simulink model "OpenMan"  (R2018a)
settings: Solver=ode5  StartTime=0.0  StopTime=T  FixedStep=0.02  RelTol=1e-3
undefined symbols (not defined in the file or in its folder): Base, Link1, Link2, Link3, Link4, OpenMan, RootPart
libraries: mblibv1 x18, simulink x4
settings Model: Creator=Administrator  LastModifiedBy=Hungs
settings CodeAppCC: StateflowObjectComments=on
settings SimscapeCC: SimscapeNormalizeSystem=off
settings SimMechanicsCC: VisOnUpdateDiagram=on  VisDuringSimulation=on

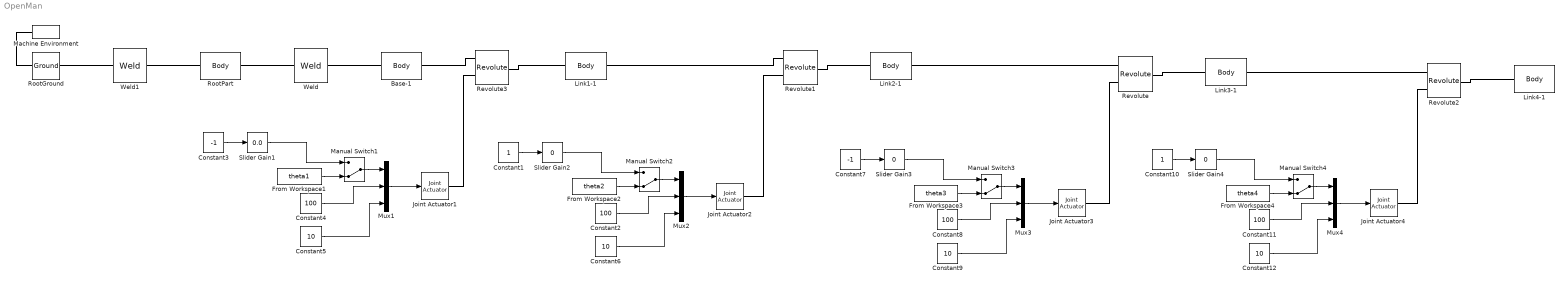
== system OpenMan ==
  Base-1 : mblibv1/Bodies/Body  LConnTagsString=CS2  RConnTagsString=CS3  UpdateFromCAD=on  PMImportedID=Base-1  DialogClass=MechanicalBodyBlock  Mass=0.0428629  MassUnits=kg  InertiaUnits=kg*m^2  Inertia=[6.81332e-06,0,-9.39051e-08;0,1.19906e-05,0;-9.39051e-08,0,1.05921e-05]  Shape=Cylinder  ShapeDims=[1 1]  ShapeUnits=m  ShapeUse=false  Density=1  DensityUnits=kg/m^3  DensityUse=false  GraphicsMode=GFXFILE  GraphicsFileName=OpenMan - Base-1.STL  BodyColorSelMode=COLORPALETTE  BodyColor=[0.64706;0.61961;0.58823]  AttachedToCS=CS1  CG=Right$CG$[-0.0116952 0 0.017999]$WORLD$WORLD$m$[1 0 0;0 1 0;0 0 1]$3x3 Transform$rad$WORLD$false$Base-1::CG(AUTOGEN)  WorkingFrames=Right$CS1$[0 0 0]$WORLD$WORLD$m$[1 0 0;0 1 0;0 0 1]$3x3 Transform$rad$WORLD$false$Base-1::CS1(AUTOGEN)#Left$CS2$[-0.0116952 0 0.017999]$WORLD$WORLD$m$[1 0 0;0 1 0;0 0 1]$3x3 Transform$rad$WORLD$true$Base-1:-:OpenMan/RootPart::Base-1(AUTOGEN)#Right$CS3$[0 0 0.036]$WORLD$WORLD$m$[1 0 0;0 1 0;0 0 1]$3x3 Transform$rad$WORLD$true$Base-1:-:Link1-1::Base-1(AUTOGEN)  CGPos=[-0.0116952 0 0.017999]  CGRot=[1 0 0;0 1 0;0 0 1]  CS0Pos=[]  CS0Rot=[]  CS1Pos=[0 0 0]  CS1Rot=[1 0 0;0 1 0;0 0 1]  CS2Pos=[-0.0116952 0 0.017999]  CS2Rot=[1 0 0;0 1 0;0 0 1]  CS3Pos=[0 0 0.036]  CS3Rot=[1 0 0;0 1 0;0 0 1]  CS4Pos=[]  CS4Rot=[]  CS5Pos=[]  CS5Rot=[]  CS6Pos=[]  CS6Rot=[]  CS7Pos=[]  CS7Rot=[]  CS8Pos=[]  CS8Rot=[]  CS9Pos=[]  CS9Rot=[]  CS10Pos=[]  CS10Rot=[]  CS11Pos=[]  CS11Rot=[]  CS12Pos=[]  CS12Rot=[]  CS13Pos=[]  CS13Rot=[]  CS14Pos=[]  CS14Rot=[]  CS15Pos=[]  CS15Rot=[]  CS16Pos=[]  CS16Rot=[]  CS17Pos=[]  CS17Rot=[]  CS18Pos=[]  CS18Rot=[]  CS19Pos=[]  CS19Rot=[]  CS20Pos=[]  CS20Rot=[]
      settings: SourceProductName=Simscape Multibody  SourceProductBaseCode=MS
  Constant1 : Constant
  Constant10 : Constant
  Constant{2,4,8,11} (4 alike) : Constant  Value=100
  Constant{5..6,9,12} (4 alike) : Constant  Value=10
  Constant3 : Constant  Value=-1
  Constant7 : Constant  Value=-1
  From Workspace1 : FromWorkspace  VariableName=theta1  SampleTime=0  OutputAfterFinalValue=Holding final value
  From Workspace2 : FromWorkspace  VariableName=theta2  SampleTime=0  OutputAfterFinalValue=Holding final value
  From Workspace3 : FromWorkspace  VariableName=theta3  SampleTime=0  OutputAfterFinalValue=Holding final value
  From Workspace4 : FromWorkspace  VariableName=theta4  SampleTime=0  OutputAfterFinalValue=Holding final value
  Joint Actuator{1..4} (4 alike) : mblibv1/Sensors &  Actuators/Joint Actuator  UpdateFromCAD=off  PhysicalDomain=Mechanical  PortType=blob  ActuationStyle=Motion  AngleUnits=deg  ArcVelocityUnits=deg/s  ArcAccelerationUnits=deg/s^2  CoordPositionUnits=m  VelocityUnits=m/s  AccelerationUnits=m/s^2  ForceUnits=N  TorqueUnits=N*m  ActiveIO=on  Width=3  DialogClass=MechanicalActuatorBlock  Primitive=R1  ReferenceFrame=Absolute (World)
      settings: SourceProductName=Simscape  SourceProductBaseCode=SS
  Link1-1 : mblibv1/Bodies/Body  LConnTagsString=CS3  RConnTagsString=CS2  UpdateFromCAD=on  PMImportedID=Link1-1  DialogClass=MechanicalBodyBlock  Mass=0.0553342  MassUnits=kg  InertiaUnits=kg*m^2  Inertia=[1.8235e-05,0,0;0,1.05975e-05,0;0,0,1.53152e-05]  Shape=Cylinder  ShapeDims=[1 1]  ShapeUnits=m  ShapeUse=false  Density=1  DensityUnits=kg/m^3  DensityUse=false  GraphicsMode=GFXFILE  GraphicsFileName=OpenMan - Link1-1.STL  BodyColorSelMode=COLORPALETTE  BodyColor=[0;1;0]  AttachedToCS=CS1  CG=Right$CG$[0 0 0.05625]$WORLD$WORLD$m$[1 0 0;0 0 -1;0 1 0]$3x3 Transform$rad$WORLD$false$Link1-1::CG(AUTOGEN)  WorkingFrames=Right$CS1$[0 0 0.0765]$WORLD$WORLD$m$[1 0 0;0 0 -1;0 1 0]$3x3 Transform$rad$WORLD$false$Link1-1::CS1(AUTOGEN)#Right$CS2$[0 0.019 0.0765]$WORLD$WORLD$m$[1 0 0;0 1 0;0 0 1]$3x3 Transform$rad$WORLD$true$Link1-1:-:Link2-1::Link1-1(AUTOGEN)#Left$CS3$[0 0 0.036]$WORLD$WORLD$m$[1 0 0;0 1 0;0 0 1]$3x3 Transform$rad$WORLD$true$Base-1:-:Link1-1::Link1-1(AUTOGEN)  CGPos=[0 0 0.05625]  CGRot=[1 0 0;0 0 -1;0 1 0]  CS0Pos=[]  CS0Rot=[]  CS1Pos=[0 0 0.0765]  CS1Rot=[1 0 0;0 0 -1;0 1 0]  CS2Pos=[0 0.019 0.0765]  CS2Rot=[1 0 0;0 1 0;0 0 1]  CS3Pos=[0 0 0.036]  CS3Rot=[1 0 0;0 1 0;0 0 1]  CS4Pos=[]  CS4Rot=[]  CS5Pos=[]  CS5Rot=[]  CS6Pos=[]  CS6Rot=[]  CS7Pos=[]  CS7Rot=[]  CS8Pos=[]  CS8Rot=[]  CS9Pos=[]  CS9Rot=[]  CS10Pos=[]  CS10Rot=[]  CS11Pos=[]  CS11Rot=[]  CS12Pos=[]  CS12Rot=[]  CS13Pos=[]  CS13Rot=[]  CS14Pos=[]  CS14Rot=[]  CS15Pos=[]  CS15Rot=[]  CS16Pos=[]  CS16Rot=[]  CS17Pos=[]  CS17Rot=[]  CS18Pos=[]  CS18Rot=[]  CS19Pos=[]  CS19Rot=[]  CS20Pos=[]  CS20Rot=[]
      settings: SourceProductName=Simscape Multibody  SourceProductBaseCode=MS
  Link2-1 : mblibv1/Bodies/Body  LConnTagsString=CS3  RConnTagsString=CS2  UpdateFromCAD=on  PMImportedID=Link2-1  DialogClass=MechanicalBodyBlock  Mass=0.117048  MassUnits=kg  InertiaUnits=kg*m^2  Inertia=[0.000233359,-2.83101e-05,0;-2.83101e-05,3.2542e-05,0;0,0,0.00023539]  Shape=Cylinder  ShapeDims=[1 1]  ShapeUnits=m  ShapeUse=false  Density=1  DensityUnits=kg/m^3  DensityUse=false  GraphicsMode=GFXFILE  GraphicsFileName=OpenMan - Link2-1.STL  BodyColorSelMode=COLORPALETTE  BodyColor=[1;1;0]  AttachedToCS=CS1  CG=Right$CG$[0.012 0 0.1405]$WORLD$WORLD$m$[1 0 0;0 0 -1;0 1 0]$3x3 Transform$rad$WORLD$false$Link2-1::CG(AUTOGEN)  WorkingFrames=Right$CS1$[0.024 0 0.2045]$WORLD$WORLD$m$[1 0 0;0 0 -1;0 1 0]$3x3 Transform$rad$WORLD$false$Link2-1::CS1(AUTOGEN)#Right$CS2$[0.024 -0.019 0.2045]$WORLD$WORLD$m$[1 0 0;0 1 0;0 0 1]$3x3 Transform$rad$WORLD$true$Link2-1:-:Link3-1::Link2-1(AUTOGEN)#Left$CS3$[0 0.019 0.0765]$WORLD$WORLD$m$[1 0 0;0 1 0;0 0 1]$3x3 Transform$rad$WORLD$true$Link1-1:-:Link2-1::Link2-1(AUTOGEN)  CGPos=[0.012 0 0.1405]  CGRot=[1 0 0;0 0 -1;0 1 0]  CS0Pos=[]  CS0Rot=[]  CS1Pos=[0.024 0 0.2045]  CS1Rot=[1 0 0;0 0 -1;0 1 0]  CS2Pos=[0.024 -0.019 0.2045]  CS2Rot=[1 0 0;0 1 0;0 0 1]  CS3Pos=[0 0.019 0.0765]  CS3Rot=[1 0 0;0 1 0;0 0 1]  CS4Pos=[]  CS4Rot=[]  CS5Pos=[]  CS5Rot=[]  CS6Pos=[]  CS6Rot=[]  CS7Pos=[]  CS7Rot=[]  CS8Pos=[]  CS8Rot=[]  CS9Pos=[]  CS9Rot=[]  CS10Pos=[]  CS10Rot=[]  CS11Pos=[]  CS11Rot=[]  CS12Pos=[]  CS12Rot=[]  CS13Pos=[]  CS13Rot=[]  CS14Pos=[]  CS14Rot=[]  CS15Pos=[]  CS15Rot=[]  CS16Pos=[]  CS16Rot=[]  CS17Pos=[]  CS17Rot=[]  CS18Pos=[]  CS18Rot=[]  CS19Pos=[]  CS19Rot=[]  CS20Pos=[]  CS20Rot=[]
      settings: SourceProductName=Simscape Multibody  SourceProductBaseCode=MS
  Link3-1 : mblibv1/Bodies/Body  LConnTagsString=CS2  RConnTagsString=CS3  UpdateFromCAD=on  PMImportedID=Link3-1  DialogClass=MechanicalBodyBlock  Mass=0.0869839  MassUnits=kg  InertiaUnits=kg*m^2  Inertia=[1.69409e-05,0,0;0,0.000140539,0;0,0,0.000129904]  Shape=Cylinder  ShapeDims=[1 1]  ShapeUnits=m  ShapeUse=false  Density=1  DensityUnits=kg/m^3  DensityUse=false  GraphicsMode=GFXFILE  GraphicsFileName=OpenMan - Link3-1.STL  BodyColorSelMode=COLORPALETTE  BodyColor=[0;0;1]  AttachedToCS=CS1  CG=Right$CG$[0.086 0 0.2045]$WORLD$WORLD$m$[1 0 0;0 0 -1;0 1 0]$3x3 Transform$rad$WORLD$false$Link3-1::CG(AUTOGEN)  WorkingFrames=Right$CS1$[0.148 0 0.2045]$WORLD$WORLD$m$[1 0 0;0 0 -1;0 1 0]$3x3 Transform$rad$WORLD$false$Link3-1::CS1(AUTOGEN)#Left$CS2$[0.024 -0.019 0.2045]$WORLD$WORLD$m$[1 0 0;0 1 0;0 0 1]$3x3 Transform$rad$WORLD$true$Link2-1:-:Link3-1::Link3-1(AUTOGEN)#Right$CS3$[0.148 0.019 0.2045]$WORLD$WORLD$m$[1 0 0;0 1 0;0 0 1]$3x3 Transform$rad$WORLD$true$Link3-1:-:Link4-1::Link3-1(AUTOGEN)  CGPos=[0.086 0 0.2045]  CGRot=[1 0 0;0 0 -1;0 1 0]  CS0Pos=[]  CS0Rot=[]  CS1Pos=[0.148 0 0.2045]  CS1Rot=[1 0 0;0 0 -1;0 1 0]  CS2Pos=[0.024 -0.019 0.2045]  CS2Rot=[1 0 0;0 1 0;0 0 1]  CS3Pos=[0.148 0.019 0.2045]  CS3Rot=[1 0 0;0 1 0;0 0 1]  CS4Pos=[]  CS4Rot=[]  CS5Pos=[]  CS5Rot=[]  CS6Pos=[]  CS6Rot=[]  CS7Pos=[]  CS7Rot=[]  CS8Pos=[]  CS8Rot=[]  CS9Pos=[]  CS9Rot=[]  CS10Pos=[]  CS10Rot=[]  CS11Pos=[]  CS11Rot=[]  CS12Pos=[]  CS12Rot=[]  CS13Pos=[]  CS13Rot=[]  CS14Pos=[]  CS14Rot=[]  CS15Pos=[]  CS15Rot=[]  CS16Pos=[]  CS16Rot=[]  CS17Pos=[]  CS17Rot=[]  CS18Pos=[]  CS18Rot=[]  CS19Pos=[]  CS19Rot=[]  CS20Pos=[]  CS20Rot=[]
      settings: SourceProductName=Simscape Multibody  SourceProductBaseCode=MS
  Link4-1 : mblibv1/Bodies/Body  LConnTagsString=CS2  UpdateFromCAD=on  PMImportedID=Link4-1  DialogClass=MechanicalBodyBlock  Mass=0.16348  MassUnits=kg  InertiaUnits=kg*m^2  Inertia=[0.000112546,0,0;0,0.000266976,0;0,0,0.000183011]  Shape=Cylinder  ShapeDims=[1 1]  ShapeUnits=m  ShapeUse=false  Density=1  DensityUnits=kg/m^3  DensityUse=false  GraphicsMode=GFXFILE  GraphicsFileName=OpenMan - Link4-1.STL  BodyColorSelMode=COLORPALETTE  BodyColor=[1 0 0]  AttachedToCS=CS1  CG=Right$CG$[0.211 0 0.2045]$WORLD$WORLD$m$[1 0 0;0 0 -1;0 1 0]$3x3 Transform$rad$WORLD$false$Link4-1::CG(AUTOGEN)  WorkingFrames=Right$CS1$[0.274 0 0.2045]$WORLD$WORLD$m$[1 0 0;0 0 -1;0 1 0]$3x3 Transform$rad$WORLD$false$Link4-1::CS1(AUTOGEN)#Left$CS2$[0.148 0.019 0.2045]$WORLD$WORLD$m$[1 0 0;0 1 0;0 0 1]$3x3 Transform$rad$WORLD$true$Link3-1:-:Link4-1::Link4-1(AUTOGEN)  CGPos=[0.211 0 0.2045]  CGRot=[1 0 0;0 0 -1;0 1 0]  CS0Pos=[]  CS0Rot=[]  CS1Pos=[0.274 0 0.2045]  CS1Rot=[1 0 0;0 0 -1;0 1 0]  CS2Pos=[0.148 0.019 0.2045]  CS2Rot=[1 0 0;0 1 0;0 0 1]  CS3Pos=[]  CS3Rot=[]  CS4Pos=[]  CS4Rot=[]  CS5Pos=[]  CS5Rot=[]  CS6Pos=[]  CS6Rot=[]  CS7Pos=[]  CS7Rot=[]  CS8Pos=[]  CS8Rot=[]  CS9Pos=[]  CS9Rot=[]  CS10Pos=[]  CS10Rot=[]  CS11Pos=[]  CS11Rot=[]  CS12Pos=[]  CS12Rot=[]  CS13Pos=[]  CS13Rot=[]  CS14Pos=[]  CS14Rot=[]  CS15Pos=[]  CS15Rot=[]  CS16Pos=[]  CS16Rot=[]  CS17Pos=[]  CS17Rot=[]  CS18Pos=[]  CS18Rot=[]  CS19Pos=[]  CS19Rot=[]  CS20Pos=[]  CS20Rot=[]
      settings: SourceProductName=Simscape Multibody  SourceProductBaseCode=MS
  Machine Environment : mblibv1/Bodies/Machine Environment  PortType=env  PhysicalDomain=Mechanical  DialogTemplateClass=MECH.MachineEnvironment  SyncWhenCopied=off  Gravity=[0 -9.81 0]  GravityUnits=m/s^2  GravityAsSignal=off  Dimensionality=Auto-detect  AnalysisType=Forward dynamics  LinearAssemblyTolerance=1e-3  LinearAssemblyToleranceUnits=m  AngularAssemblyTolerance=1e-3  AngularAssemblyToleranceUnits=rad  ConstraintSolverType=Stabilizing  ConstraintRelTolerance=1e-4  ConstraintAbsTolerance=1e-4  UseRobustSingularityHandling=off  RedundancyAnalysisToleranceType=Automatically select tolerance  RedundancyAnalysisTolerance=1e-14  StatePerturbationType=Fixed  PerturbationSize=1e-5  VisualizeMachine=on  BodyVisualizationType=Use model default body geometries  BodyColorSelMode=Use model default  DefaultBodyColor=[1 0 0]
      settings: SourceProductName=Simscape Multibody  SourceProductBaseCode=MS
  Manual Switch{1..4} (4 alike) : ManualSwitch  CurrentSetting=0
  Mux{1..4} (4 alike) : Mux  Inputs=3
  Revolute : mblibv1/Joints/Revolute  LConnTagsString=__newl0|SA1  RConnTagsString=__newr0  UpdateFromCAD=on  PMImportedID=Link2-1:-:Link3-1  NumSAPorts=1  CutJoint=off  MarkAsCut=off  Primitives=prismatic  PrimitiveProps=R1$World$[0,1,0]$revolute  DialogClass=JointBlock  R1Axis=[0,1,0]
      settings: SourceProductName=Simscape Multibody  SourceProductBaseCode=MS
  Revolute1 : mblibv1/Joints/Revolute  LConnTagsString=__newl0|SA1  RConnTagsString=__newr0  UpdateFromCAD=on  PMImportedID=Link1-1:-:Link2-1  NumSAPorts=1  CutJoint=off  MarkAsCut=off  Primitives=prismatic  PrimitiveProps=R1$World$[0,-1,0]$revolute  DialogClass=JointBlock  R1Axis=[0,-1,0]
      settings: SourceProductName=Simscape Multibody  SourceProductBaseCode=MS
  Revolute2 : mblibv1/Joints/Revolute  LConnTagsString=__newl0|SA1  RConnTagsString=__newr0  UpdateFromCAD=on  PMImportedID=Link3-1:-:Link4-1  NumSAPorts=1  CutJoint=off  MarkAsCut=off  Primitives=prismatic  PrimitiveProps=R1$World$[0,-1,0]$revolute  DialogClass=JointBlock  R1Axis=[0,-1,0]
      settings: SourceProductName=Simscape Multibody  SourceProductBaseCode=MS
  Revolute3 : mblibv1/Joints/Revolute  LConnTagsString=__newl0|SA1  RConnTagsString=__newr0  UpdateFromCAD=on  PMImportedID=Base-1:-:Link1-1  NumSAPorts=1  CutJoint=off  MarkAsCut=off  Primitives=prismatic  PrimitiveProps=R1$World$[0,0,-1]$revolute  DialogClass=JointBlock  R1Axis=[0,0,-1]
      settings: SourceProductName=Simscape Multibody  SourceProductBaseCode=MS
  RootGround : mblibv1/Bodies/Ground  UpdateFromCAD=on  PMImportedID=RootGround  LeftPortType=env  RightPortType=workingframe  PhysicalDomain=Mechanical  DialogClass=GroundBlock  CoordPosition=[0.219004,-0.00655955,0.163625]  CoordPositionUnits=m  StateVectorMgrId=0  MachineId=[1 0]  ShowEnvPort=on  ParameterChecksum=[2384219016, 3002916829, 4077460786, 3927882011]  TopologyChecksum=[2459791412, 654682897, 3936132905, 4259893478]
      settings: SourceProductName=Simscape Multibody  SourceProductBaseCode=MS
  RootPart : mblibv1/Bodies/Body  LConnTagsString=CS3  RConnTagsString=CS2  UpdateFromCAD=on  PMImportedID=OpenMan/RootPart  DialogClass=MechanicalBodyBlock  Mass=0  MassUnits=kg  InertiaUnits=kg*m^2  Inertia=[0,0,0;0,0,0;0,0,0]  Shape=Cylinder  ShapeDims=[1 1]  ShapeUnits=m  ShapeUse=false  Density=1  DensityUnits=kg/m^3  DensityUse=false  GraphicsMode=MACHINE_DEFAULT  BodyColorSelMode=MACHINE_DEFAULT  BodyColor=[1;0;0]  AttachedToCS=CS1  CG=Right$CG$[0.219004 -0.00655955 0.163625]$WORLD$WORLD$m$[1 0 0;0 1 0;0 0 1]$3x3 Transform$rad$WORLD$false$OpenMan/RootPart::CG(AUTOGEN)  WorkingFrames=Right$CS1$[0 0 0]$WORLD$WORLD$m$[1 0 0;0 1 0;0 0 1]$3x3 Transform$rad$WORLD$false$OpenMan/RootPart::CS1(AUTOGEN)#Right$CS2$[-0.0116952 0 0.017999]$WORLD$WORLD$m$[1 0 0;0 1 0;0 0 1]$3x3 Transform$rad$WORLD$true$Base-1:-:OpenMan/RootPart::OpenMan/RootPart(AUTOGEN)#Left$CS3$[0.219004 -0.00655955 0.163625]$WORLD$WORLD$m$[1 0 0;0 1 0;0 0 1]$3x3 Transform$rad$WORLD$true$OpenMan/RootPart:-:RootGround::OpenMan/RootPart(AUTOGEN)  CGPos=[0.219004 -0.00655955 0.163625]  CGRot=[1 0 0;0 1 0;0 0 1]  CS0Pos=[]  CS0Rot=[]  CS1Pos=[0 0 0]  CS1Rot=[1 0 0;0 1 0;0 0 1]  CS2Pos=[-0.0116952 0 0.017999]  CS2Rot=[1 0 0;0 1 0;0 0 1]  CS3Pos=[0.219004 -0.00655955 0.163625]  CS3Rot=[1 0 0;0 1 0;0 0 1]  CS4Pos=[]  CS4Rot=[]  CS5Pos=[]  CS5Rot=[]  CS6Pos=[]  CS6Rot=[]  CS7Pos=[]  CS7Rot=[]  CS8Pos=[]  CS8Rot=[]  CS9Pos=[]  CS9Rot=[]  CS10Pos=[]  CS10Rot=[]  CS11Pos=[]  CS11Rot=[]  CS12Pos=[]  CS12Rot=[]  CS13Pos=[]  CS13Rot=[]  CS14Pos=[]  CS14Rot=[]  CS15Pos=[]  CS15Rot=[]  CS16Pos=[]  CS16Rot=[]  CS17Pos=[]  CS17Rot=[]  CS18Pos=[]  CS18Rot=[]  CS19Pos=[]  CS19Rot=[]  CS20Pos=[]  CS20Rot=[]
      settings: SourceProductName=Simscape Multibody  SourceProductBaseCode=MS
  Slider Gain1 : simulink/Math Operations/Slider Gain  gain=0.0  low=-180  high=180
  Slider Gain2 : simulink/Math Operations/Slider Gain  gain=0  low=-180  high=180
  Slider Gain3 : simulink/Math Operations/Slider Gain  gain=0  low=-180  high=180
  Slider Gain4 : simulink/Math Operations/Slider Gain  gain=0  low=-180  high=180
  Weld : mblibv1/Joints/Weld  LConnTagsString=__newl0  RConnTagsString=__newr0  UpdateFromCAD=on  PMImportedID=Base-1:-:OpenMan/RootPart  NumSAPorts=0  CutJoint=off  MarkAsCut=off  Primitives=weld  PrimitiveProps=W$WORLD$[0.57735,0.57735,0.57735]$weld  DialogClass=JointBlock  WAxis=[0.57735,0.57735,0.57735]
      settings: SourceProductName=Simscape Multibody  SourceProductBaseCode=MS
  Weld1 : mblibv1/Joints/Weld  LConnTagsString=__newl0  RConnTagsString=__newr0  UpdateFromCAD=on  PMImportedID=OpenMan/RootPart:-:RootGround  NumSAPorts=0  CutJoint=off  MarkAsCut=off  Primitives=weld  PrimitiveProps=W$WORLD$[0.57735,0.57735,0.57735]$weld  DialogClass=JointBlock  WAxis=[0.57735,0.57735,0.57735]
      settings: SourceProductName=Simscape Multibody  SourceProductBaseCode=MS
  wires:
  Slider Gain1/1 -> Manual Switch1/1
  Manual Switch1/1 -> Mux1/1
  Constant3/1 -> Slider Gain1/1
  From Workspace1/1 -> Manual Switch1/2
  Constant5/1 -> Mux1/3
  Mux1/1 -> Joint Actuator1/1
  Constant4/1 -> Mux1/2
  Constant2/1 -> Mux2/2
  Manual Switch2/1 -> Mux2/1
  Constant6/1 -> Mux2/3
  Constant1/1 -> Slider Gain2/1
  From Workspace2/1 -> Manual Switch2/2
  Mux2/1 -> Joint Actuator2/1
  Slider Gain2/1 -> Manual Switch2/1
  Constant8/1 -> Mux3/2
  Manual Switch3/1 -> Mux3/1
  Constant9/1 -> Mux3/3
  Constant7/1 -> Slider Gain3/1
  From Workspace3/1 -> Manual Switch3/2
  Mux3/1 -> Joint Actuator3/1
  Slider Gain3/1 -> Manual Switch3/1
  Constant11/1 -> Mux4/2
  Manual Switch4/1 -> Mux4/1
  Constant12/1 -> Mux4/3
  Constant10/1 -> Slider Gain4/1
  From Workspace4/1 -> Manual Switch4/2
  Mux4/1 -> Joint Actuator4/1
  Slider Gain4/1 -> Manual Switch4/1
  connections:
  RootPart/RConn1 -- Weld/LConn1
  Weld/RConn1 -- Base-1/LConn1
  Link2-1/RConn1 -- Revolute/LConn1
  Revolute/RConn1 -- Link3-1/LConn1
  Link1-1/RConn1 -- Revolute1/LConn1
  Revolute1/RConn1 -- Link2-1/LConn1
  Link3-1/RConn1 -- Revolute2/LConn1
  Revolute2/RConn1 -- Link4-1/LConn1
  Base-1/RConn1 -- Revolute3/LConn1
  Revolute3/RConn1 -- Link1-1/LConn1
  RootGround/RConn1 -- Weld1/LConn1
  Weld1/RConn1 -- RootPart/LConn1
  RootGround/LConn1 -- Machine Environment/RConn1
  Joint Actuator1/RConn1 -- Revolute3/LConn2
  Joint Actuator2/RConn1 -- Revolute1/LConn2
  Joint Actuator3/RConn1 -- Revolute/LConn2
  Joint Actuator4/RConn1 -- Revolute2/LConn2
